simulink model "FastAndSlow"  (R2024b)
settings: Solver=VariableStepAuto  StartTime=0.0  StopTime=86400*2  RelTol=1e-3
values from neighbouring files (symbols this model uses):
  xk0 = zeros(36, 1)    [getinput_test.m]
(part 2 of 2)

== matlab function FastAndSlow/GP_1step ==
  data: y_model input; e_pred output; y_meas input; T input; P1 input; P2 input; P3 input; P4 input; P5 input; t input; comp_time output
function [e_pred, comp_time]= GP_onestep(y_model, y_meas, T, P1, P2, P3, P4, P5, t)
    
    % Declare we use some matlab function inside the Simulink block
    coder.extrinsic('fitrgp', 'predict')
    
    % Declare parameters
    n_regression = 4;
    sampling_time = 300;
    n_input = 6;
    n_output = size(y_model,1);
    delta_e_max = 20;
    n_max = 48; %300

    % Declare persistent variables whose dimension is not fixed (used to have an increasing dataset)
    persistent e_pers u_pers u_stack e_stack_1 e_stack_2 e_stack_3 e_stack_4 e_stack_5 e_stack_6 e_stack_7 e_stack_8 e_stack_9 e_stack_10 e_stack_11 e_stack_12 e_stack_13 e_stack_14 e_stack_15 e_stack_16 e_stack_17 e_pred_tot y_pers y_stack_1 y_stack_2 y_stack_3 y_stack_4 y_stack_5 y_stack_6 y_stack_7 y_stack_8 y_stack_9 y_stack_10 y_stack_11 y_stack_12 y_stack_13 y_stack_14 y_stack_15 y_stack_16 y_stack_17
    coder.varsize('u_pers', [inf, n_input]);
    coder.varsize('u_stack', [inf, n_input*n_regression]);
    coder.varsize('e_pred_tot', [inf, n_output]);
    coder.varsize('e_pers', [inf, n_output]);
    coder.varsize('e_stack_1', [inf, n_regression]);
    coder.varsize('e_stack_2', [inf, n_regression]);
    coder.varsize('e_stack_3', [inf, n_regression]);
    coder.varsize('e_stack_4', [inf, n_regression]);
    coder.varsize('e_stack_5', [inf, n_regression]);
    coder.varsize('e_stack_6', [inf, n_regression]);
    coder.varsize('e_stack_7', [inf, n_regression]);
    coder.varsize('e_stack_8', [inf, n_regression]);
    coder.varsize('e_stack_9', [inf, n_regression]);
    coder.varsize('e_stack_10', [inf, n_regression]);
    coder.varsize('e_stack_11', [inf, n_regression]);
    coder.varsize('e_stack_12', [inf, n_regression]);
    coder.varsize('e_stack_13', [inf, n_regression]);
    coder.varsize('e_stack_14', [inf, n_regression]);
    coder.varsize('e_stack_15', [inf, n_regression]);
    coder.varsize('e_stack_16', [inf, n_regression]);
    coder.varsize('e_stack_17', [inf, n_regression]);
    coder.varsize('y_pers', [inf, n_output]);
    coder.varsize('y_stack_1', [inf, n_regression]);
    coder.varsize('y_stack_2', [inf, n_regression]);
    coder.varsize('y_stack_3', [inf, n_regression]);
    coder.varsize('y_stack_4', [inf, n_regression]);
    coder.varsize('y_stack_5', [inf, n_regression]);
    coder.varsize('y_stack_6', [inf, n_regression]);
    coder.varsize('y_stack_7', [inf, n_regression]);
    coder.varsize('y_stack_8', [inf, n_regression]);
    coder.varsize('y_stack_9', [inf, n_regression]);
    coder.varsize('y_stack_10', [inf, n_regression]);
    coder.varsize('y_stack_11', [inf, n_regression]);
    coder.varsize('y_stack_12', [inf, n_regression]);
    coder.varsize('y_stack_13', [inf, n_regression]);
    coder.varsize('y_stack_14', [inf, n_regression]);
    coder.varsize('y_stack_15', [inf, n_regression]);
    coder.varsize('y_stack_16', [inf, n_regression]);
    coder.varsize('y_stack_17', [inf, n_regression]);
    
    % Initialize persistent variables
    if isempty(e_pers)
        u_pers = zeros(1,n_input);
        u_stack = zeros(1,n_input*n_regression);
        e_pred_tot = zeros(1,n_output);
        e_pers = zeros(1,n_output);
        e_stack_1 = zeros(1,n_regression);
        e_stack_2 = zeros(1,n_regression);
        e_stack_3 = zeros(1,n_regression);
        e_stack_4 = zeros(1,n_regression);
        e_stack_5 = zeros(1,n_regression);
        e_stack_6 = zeros(1,n_regression);
        e_stack_7 = zeros(1,n_regression);
        e_stack_8 = zeros(1,n_regression);
        e_stack_9 = zeros(1,n_regression);
        e_stack_10 = zeros(1,n_regression);
        e_stack_11 = zeros(1,n_regression);
        e_stack_12 = zeros(1,n_regression);
        e_stack_13 = zeros(1,n_regression);
        e_stack_14 = zeros(1,n_regression);
        e_stack_15 = zeros(1,n_regression);
        e_stack_16 = zeros(1,n_regression);
        e_stack_17 = zeros(1,n_regression);
        y_pers = zeros(1,n_output);
        y_stack_1 = zeros(1,n_regression);
        y_stack_2 = zeros(1,n_regression);
        y_stack_3 = zeros(1,n_regression);
        y_stack_4 = zeros(1,n_regression);
        y_stack_5 = zeros(1,n_regression);
        y_stack_6 = zeros(1,n_regression);
        y_stack_7 = zeros(1,n_regression);
        y_stack_8 = zeros(1,n_regression);
        y_stack_9 = zeros(1,n_regression);
        y_stack_10 = zeros(1,n_regression);
        y_stack_11 = zeros(1,n_regression);
        y_stack_12 = zeros(1,n_regression);
        y_stack_13 = zeros(1,n_regression);
        y_stack_14 = zeros(1,n_regression);
        y_stack_15 = zeros(1,n_regression);
        y_stack_16 = zeros(1,n_regression);
        y_stack_17 = zeros(1,n_regression);
    end
    
    % Output initialization
    e_pred = zeros(17,1);

    % Create increasing input dataset
    u_new = [T P1 P2 P3 P4 P5];
    u_pers = [u_pers; u_new];
    
    % Create increasing uncertainty dataset
    y_meas = [y_meas(1); y_meas(6); y_meas(11); y_meas(4); y_meas(9); y_meas(14); y_meas(2); y_meas(7); y_meas(12); y_meas(3); y_meas(8); y_meas(13); y_meas(5); y_meas(10); y_meas(15); y_meas(16); y_meas(17)];
    e_new = (y_meas - y_model).';
    e_pers = [e_pers; e_new];

    % Create increasing y model dataset
    y_pers = [y_pers; y_model.'];
    
    % Remove first row of zeros
    if e_pers(1,1) == 0
        u_pers = u_pers(2:end,:);
        e_pers = e_pers(2:end,:);
        y_pers = y_pers(2:end,:);
    end
    
    comp_time = 0;
    
    % Start to build GP when data are at least n_regression
    if t >= sampling_time*n_regression
        
        tic

        % Build the regressive variables
        u_regr = zeros(1,size(u_stack,2));
        u_regr_test = zeros(1,size(u_stack,2));
        k = 1;
        for i = 1:n_regression
            u_regr(1,k:k+n_input-1) = u_pers(end-i,:);
            u_regr_test(1,k:k+n_input-1) = u_pers(end-i+1,:);
            k = k + n_input;
        end

        e_regr_1 = zeros(1,size(e_stack_1,2));
        e_regr_1_test = zeros(1,size(e_stack_1,2));
        e_regr_2 = zeros(1,size(e_stack_2,2));
        e_regr_2_test = zeros(1,size(e_stack_2,2));
        e_regr_3 = zeros(1,size(e_stack_3,2));
        e_regr_3_test = zeros(1,size(e_stack_3,2));
        e_regr_4 = zeros(1,size(e_stack_4,2));
        e_regr_4_test = zeros(1,size(e_stack_4,2));
        e_regr_5 = zeros(1,size(e_stack_5,2));
        e_regr_5_test = zeros(1,size(e_stack_5,2));
        e_regr_6 = zeros(1,size(e_stack_6,2));
        e_regr_6_test = zeros(1,size(e_stack_6,2));
        e_regr_7 = zeros(1,size(e_stack_7,2));
        e_regr_7_test = zeros(1,size(e_stack_7,2));
        e_regr_8 = zeros(1,size(e_stack_8,2));
        e_regr_8_test = zeros(1,size(e_stack_8,2));
        e_regr_9 = zeros(1,size(e_stack_9,2));
        e_regr_9_test = zeros(1,size(e_stack_9,2));
        e_regr_10 = zeros(1,size(e_stack_10,2));
        e_regr_10_test = zeros(1,size(e_stack_10,2));
        e_regr_11 = zeros(1,size(e_stack_11,2));
        e_regr_11_test = zeros(1,size(e_stack_11,2));
        e_regr_12 = zeros(1,size(e_stack_12,2));
        e_regr_12_test = zeros(1,size(e_stack_12,2));
        e_regr_13 = zeros(1,size(e_stack_13,2));
        e_regr_13_test = zeros(1,size(e_stack_13,2));
        e_regr_14 = zeros(1,size(e_stack_14,2));
        e_regr_14_test = zeros(1,size(e_stack_14,2));
        e_regr_15 = zeros(1,size(e_stack_15,2));
        e_regr_15_test = zeros(1,size(e_stack_15,2));
        e_regr_16 = zeros(1,size(e_stack_16,2));
        e_regr_16_test = zeros(1,size(e_stack_16,2));
        e_regr_17 = zeros(1,size(e_stack_17,2));
        e_regr_17_test = zeros(1,size(e_stack_17,2));
        y_regr_1 = zeros(1,size(y_stack_1,2));
        y_regr_1_test = zeros(1,size(y_stack_1,2));
        y_regr_2 = zeros(1,size(y_stack_2,2));
        y_regr_2_test = zeros(1,size(y_stack_2,2));
        y_regr_3 = zeros(1,size(y_stack_3,2));
        y_regr_3_test = zeros(1,size(y_stack_3,2));
        y_regr_4 = zeros(1,size(y_stack_4,2));
        y_regr_4_test = zeros(1,size(y_stack_4,2));
        y_regr_5 = zeros(1,size(y_stack_5,2));
        y_regr_5_test = zeros(1,size(y_stack_5,2));
        y_regr_6 = zeros(1,size(y_stack_6,2));
        y_regr_6_test = zeros(1,size(y_stack_6,2));
        y_regr_7 = zeros(1,size(y_stack_7,2));
        y_regr_7_test = zeros(1,size(y_stack_7,2));
        y_regr_8 = zeros(1,size(y_stack_8,2));
        y_regr_8_test = zeros(1,size(y_stack_8,2));
        y_regr_9 = zeros(1,size(y_stack_9,2));
        y_regr_9_test = zeros(1,size(y_stack_9,2));
        y_regr_10 = zeros(1,size(y_stack_10,2));
        y_regr_10_test = zeros(1,size(y_stack_10,2));
        y_regr_11 = zeros(1,size(y_stack_11,2));
        y_regr_11_test = zeros(1,size(y_stack_11,2));
        y_regr_12 = zeros(1,size(y_stack_12,2));
        y_regr_12_test = zeros(1,size(y_stack_12,2));
        y_regr_13 = zeros(1,size(y_stack_13,2));
        y_regr_13_test = zeros(1,size(y_stack_13,2));
        y_regr_14 = zeros(1,size(y_stack_14,2));
        y_regr_14_test = zeros(1,size(y_stack_14,2));
        y_regr_15 = zeros(1,size(y_stack_15,2));
        y_regr_15_test = zeros(1,size(y_stack_15,2));
        y_regr_16 = zeros(1,size(y_stack_16,2));
        y_regr_16_test = zeros(1,size(y_stack_16,2));
        y_regr_17 = zeros(1,size(y_stack_17,2));
        y_regr_17_test = zeros(1,size(y_stack_17,2));

        for i = 1:n_regression
            e_regr_1(1,i) = e_pers(end-i,1);
            e_regr_1_test(1,i) = e_pers(end-i+1,1);
            e_regr_2(1,i) = e_pers(end-i,2);
            e_regr_2_test(1,i) = e_pers(end-i+1,2);
            e_regr_3(1,i) = e_pers(end-i,3);
            e_regr_3_test(1,i) = e_pers(end-i+1,3);
            e_regr_4(1,i) = e_pers(end-i,4);
            e_regr_4_test(1,i) = e_pers(end-i+1,4);
            e_regr_5(1,i) = e_pers(end-i,5);
            e_regr_5_test(1,i) = e_pers(end-i+1,5);
            e_regr_6(1,i) = e_pers(end-i,6);
            e_regr_6_test(1,i) = e_pers(end-i+1,6);
            e_regr_7(1,i) = e_pers(end-i,7);
            e_regr_7_test(1,i) = e_pers(end-i+1,7);
            e_regr_8(1,i) = e_pers(end-i,8);
            e_regr_8_test(1,i) = e_pers(end-i+1,8);
            e_regr_9(1,i) = e_pers(end-i,9);
            e_regr_9_test(1,i) = e_pers(end-i+1,9);
            e_regr_10(1,i) = e_pers(end-i,10);
            e_regr_10_test(1,i) = e_pers(end-i+1,10);
            e_regr_11(1,i) = e_pers(end-i,11);
            e_regr_11_test(1,i) = e_pers(end-i+1,11);
            e_regr_12(1,i) = e_pers(end-i,12);
            e_regr_12_test(1,i) = e_pers(end-i+1,12);
            e_regr_13(1,i) = e_pers(end-i,13);
            e_regr_13_test(1,i) = e_pers(end-i+1,13);
            e_regr_14(1,i) = e_pers(end-i,14);
            e_regr_14_test(1,i) = e_pers(end-i+1,14);
            e_regr_15(1,i) = e_pers(end-i,15);
            e_regr_15_test(1,i) = e_pers(end-i+1,15);
            e_regr_16(1,i) = e_pers(end-i,16);
            e_regr_16_test(1,i) = e_pers(end-i+1,16);
            e_regr_17(1,i) = e_pers(end-i,17);
            e_regr_17_test(1,i) = e_pers(end-i+1,17);
            y_regr_1(1,i) = y_pers(end-i,1);
            y_regr_1_test(1,i) = y_pers(end-i+1,1);
            y_regr_2(1,i) = y_pers(end-i,2);
            y_regr_2_test(1,i) = y_pers(end-i+1,2);
            y_regr_3(1,i) = y_pers(end-i,3);
            y_regr_3_test(1,i) = y_pers(end-i+1,3);
            y_regr_4(1,i) = y_pers(end-i,4);
            y_regr_4_test(1,i) = y_pers(end-i+1,4);
            y_regr_5(1,i) = y_pers(end-i,5);
            y_regr_5_test(1,i) = y_pers(end-i+1,5);
            y_regr_6(1,i) = y_pers(end-i,6);
            y_regr_6_test(1,i) = y_pers(end-i+1,6);
            y_regr_7(1,i) = y_pers(end-i,7);
            y_regr_7_test(1,i) = y_pers(end-i+1,7);
            y_regr_8(1,i) = y_pers(end-i,8);
            y_regr_8_test(1,i) = y_pers(end-i+1,8);
            y_regr_9(1,i) = y_pers(end-i,9);
            y_regr_9_test(1,i) = y_pers(end-i+1,9);
            y_regr_10(1,i) = y_pers(end-i,10);
            y_regr_10_test(1,i) = y_pers(end-i+1,10);
            y_regr_11(1,i) = y_pers(end-i,11);
            y_regr_11_test(1,i) = y_pers(end-i+1,11);
            y_regr_12(1,i) = y_pers(end-i,12);
            y_regr_12_test(1,i) = y_pers(end-i+1,12);
            y_regr_13(1,i) = y_pers(end-i,13);
            y_regr_13_test(1,i) = y_pers(end-i+1,13);
            y_regr_14(1,i) = y_pers(end-i,14);
            y_regr_14_test(1,i) = y_pers(end-i+1,14);
            y_regr_15(1,i) = y_pers(end-i,15);
            y_regr_15_test(1,i) = y_pers(end-i+1,15);
            y_regr_16(1,i) = y_pers(end-i,16);
            y_regr_16_test(1,i) = y_pers(end-i+1,16);
            y_regr_17(1,i) = y_pers(end-i,17);
            y_regr_17_test(1,i) = y_pers(end-i+1,17);
        end
    
        % Stack vertically
        u_stack = [u_stack; u_regr];
        e_stack_1 = [e_stack_1; e_regr_1];
        e_stack_2 = [e_stack_2; e_regr_2];
        e_stack_3 = [e_stack_3; e_regr_3];
        e_stack_4 = [e_stack_4; e_regr_4];
        e_stack_5 = [e_stack_5; e_regr_5];
        e_stack_6 = [e_stack_6; e_regr_6];
        e_stack_7 = [e_stack_7; e_regr_7];
        e_stack_8 = [e_stack_8; e_regr_8];
        e_stack_9 = [e_stack_9; e_regr_9];
        e_stack_10 = [e_stack_10; e_regr_10];
        e_stack_11 = [e_stack_11; e_regr_11];
        e_stack_12 = [e_stack_12; e_regr_12];
        e_stack_13 = [e_stack_13; e_regr_13];
        e_stack_14 = [e_stack_14; e_regr_14];
        e_stack_15 = [e_stack_15; e_regr_15];
        e_stack_16 = [e_stack_16; e_regr_16];
        e_stack_17 = [e_stack_17; e_regr_17];
        y_stack_1 = [y_stack_1; y_regr_1];
        y_stack_2 = [y_stack_2; y_regr_2];
        y_stack_3 = [y_stack_3; y_regr_3];
        y_stack_4 = [y_stack_4; y_regr_4];
        y_stack_5 = [y_stack_5; y_regr_5];
        y_stack_6 = [y_stack_6; y_regr_6];
        y_stack_7 = [y_stack_7; y_regr_7];
        y_stack_8 = [y_stack_8; y_regr_8];
        y_stack_9 = [y_stack_9; y_regr_9];
        y_stack_10 = [y_stack_10; y_regr_10];
        y_stack_11 = [y_stack_11; y_regr_11];
        y_stack_12 = [y_stack_12; y_regr_12];
        y_stack_13 = [y_stack_13; y_regr_13];
        y_stack_14 = [y_stack_14; y_regr_14];
        y_stack_15 = [y_stack_15; y_regr_15];
        y_stack_16 = [y_stack_16; y_regr_16];
        y_stack_17 = [y_stack_17; y_regr_17];
        
        %%%%%%%%%% Input of GP %%%%%%%%%%
        % x_1 = [e_stack_1 y_stack_1 u_stack];
        % x_2 = [e_stack_2 y_stack_2 u_stack];
        % x_3 = [e_stack_3 y_stack_3 u_stack];
        % x_4 = [e_stack_4 y_stack_4 u_stack];
        % x_5 = [e_stack_5 y_stack_5 u_stack];
        % x_6 = [e_stack_6 y_stack_6 u_stack];
        % x_7 = [e_stack_7 y_stack_7 u_stack];
        % x_8 = [e_stack_8 y_stack_8 u_stack];
        % x_9 = [e_stack_9 y_stack_9 u_stack];
        % x_10 = [e_stack_10 y_stack_10 u_stack];
        % x_11 = [e_stack_11 y_stack_11 u_stack];
        % x_12 = [e_stack_12 y_stack_12 u_stack];
        % x_13 = [e_stack_13 y_stack_13 u_stack];
        % x_14 = [e_stack_14 y_stack_14 u_stack];
        % x_15 = [e_stack_15 y_stack_15 u_stack];
        % x_16 = [e_stack_16 y_stack_16 u_stack];
        % x_17 = [e_stack_17 y_stack_17 u_stack];

        x_1 = [e_stack_1 y_stack_1];
        x_2 = [e_stack_2 y_stack_2];
        x_3 = [e_stack_3 y_stack_3];
        x_4 = [e_stack_4 y_stack_4];
        x_5 = [e_stack_5 y_stack_5];
        x_6 = [e_stack_6 y_stack_6];
        x_7 = [e_stack_7 y_stack_7];
        x_8 = [e_stack_8 y_stack_8];
        x_9 = [e_stack_9 y_stack_9];
        x_10 = [e_stack_10 y_stack_10];
        x_11 = [e_stack_11 y_stack_11];
        x_12 = [e_stack_12 y_stack_12];
        x_13 = [e_stack_13 y_stack_13];
        x_14 = [e_stack_14 y_stack_14];
        x_15 = [e_stack_15 y_stack_15];
        x_16 = [e_stack_16 y_stack_16];
        x_17 = [e_stack_17 y_stack_17];

        %%%%%%%%%% GP model learning, for each output %%%%%%%%%%
        gpr_model1 = fitrgp(x_1, e_pers(n_regression:end,1));
        gpr_model2 = fitrgp(x_2, e_pers(n_regression:end,2));
        gpr_model3 = fitrgp(x_3, e_pers(n_regression:end,3));
        gpr_model4 = fitrgp(x_4, e_pers(n_regression:end,4));
        gpr_model5 = fitrgp(x_5, e_pers(n_regression:end,5));
        gpr_model6 = fitrgp(x_6, e_pers(n_regression:end,6));
        gpr_model7 = fitrgp(x_7, e_pers(n_regression:end,7));
        gpr_model8 = fitrgp(x_8, e_pers(n_regression:end,8));
        gpr_model9 = fitrgp(x_9, e_pers(n_regression:end,9));
        gpr_model10 = fitrgp(x_10, e_pers(n_regression:end,10));
        gpr_model11 = fitrgp(x_11, e_pers(n_regression:end,11));
        gpr_model12 = fitrgp(x_12, e_pers(n_regression:end,12));
        gpr_model13 = fitrgp(x_13, e_pers(n_regression:end,13));
        gpr_model14 = fitrgp(x_14, e_pers(n_regression:end,14));
        gpr_model15 = fitrgp(x_15, e_pers(n_regression:end,15));
        gpr_model16 = fitrgp(x_16, e_pers(n_regression:end,16));
        gpr_model17 = fitrgp(x_17, e_pers(n_regression:end,17));
        
        %%%%%%%%%% GP prediction %%%%%%%%%%
        % e_pred(1) = predict(gpr_model1, [e_regr_1_test y_regr_1_test u_regr_test]);
        % e_pred(2) = predict(gpr_model2, [e_regr_2_test y_regr_2_test u_regr_test]);
        % e_pred(3) = predict(gpr_model3, [e_regr_3_test y_regr_3_test u_regr_test]);
        % e_pred(4) = predict(gpr_model4, [e_regr_4_test y_regr_4_test u_regr_test]);
        % e_pred(5) = predict(gpr_model5, [e_regr_5_test y_regr_5_test u_regr_test]);
        % e_pred(6) = predict(gpr_model6, [e_regr_6_test y_regr_6_test u_regr_test]);
        % e_pred(7) = predict(gpr_model7, [e_regr_7_test y_regr_7_test u_regr_test]);
        % e_pred(8) = predict(gpr_model8, [e_regr_8_test y_regr_8_test u_regr_test]);
        % e_pred(9) = predict(gpr_model9, [e_regr_9_test y_regr_9_test u_regr_test]);
        % e_pred(10) = predict(gpr_model10, [e_regr_10_test y_regr_10_test u_regr_test]);
        % e_pred(11) = predict(gpr_model11, [e_regr_11_test y_regr_11_test u_regr_test]);
        % e_pred(12) = predict(gpr_model12, [e_regr_12_test y_regr_12_test u_regr_test]);
        % e_pred(13) = predict(gpr_model13, [e_regr_13_test y_regr_13_test u_regr_test]);
        % e_pred(14) = predict(gpr_model14, [e_regr_14_test y_regr_14_test u_regr_test]);
        % e_pred(15) = predict(gpr_model15, [e_regr_15_test y_regr_15_test u_regr_test]);
        % e_pred(16) = predict(gpr_model16, [e_regr_16_test y_regr_16_test u_regr_test]);
        % e_pred(17) = predict(gpr_model17, [e_regr_17_test y_regr_17_test u_regr_test]);

        e_pred(1) = predict(gpr_model1, [e_regr_1_test y_regr_1_test]);
        e_pred(2) = predict(gpr_model2, [e_regr_2_test y_regr_2_test]);
        e_pred(3) = predict(gpr_model3, [e_regr_3_test y_regr_3_test]);
        e_pred(4) = predict(gpr_model4, [e_regr_4_test y_regr_4_test]);
        e_pred(5) = predict(gpr_model5, [e_regr_5_test y_regr_5_test]);
        e_pred(6) = predict(gpr_model6, [e_regr_6_test y_regr_6_test]);
        e_pred(7) = predict(gpr_model7, [e_regr_7_test y_regr_7_test]);
        e_pred(8) = predict(gpr_model8, [e_regr_8_test y_regr_8_test]);
        e_pred(9) = predict(gpr_model9, [e_regr_9_test y_regr_9_test]);
        e_pred(10) = predict(gpr_model10, [e_regr_10_test y_regr_10_test]);
        e_pred(11) = predict(gpr_model11, [e_regr_11_test y_regr_11_test]);
        e_pred(12) = predict(gpr_model12, [e_regr_12_test y_regr_12_test]);
        e_pred(13) = predict(gpr_model13, [e_regr_13_test y_regr_13_test]);
        e_pred(14) = predict(gpr_model14, [e_regr_14_test y_regr_14_test]);
        e_pred(15) = predict(gpr_model15, [e_regr_15_test y_regr_15_test]);
        e_pred(16) = predict(gpr_model16, [e_regr_16_test y_regr_16_test]);
        e_pred(17) = predict(gpr_model17, [e_regr_17_test y_regr_17_test]);

        
        %%%%%%%%%% Limit the difference of the uncertainty between two consecutive time instants %%%%%%%%%%
        for i = 1:n_output
            if abs(e_pred_tot(end,i)-e_pred(i)) > delta_e_max
                e_pred(i) = e_pred_tot(end,i);
            end
        end
       
        e_pred_tot = [e_pred_tot; e_pred.'];
    
        %%%%%%%%%% Limit the size of GP %%%%%%%%%%
        if size(u_stack,1) > n_max
            u_stack = u_stack(end-n_max:end,:);
            u_pers = u_pers(end-n_max-n_regression+1:end,:);
            e_pred_tot = e_pred_tot(end-n_max:end,:);
            e_pers = e_pers(end-n_max-n_regression+1:end,:);
            e_stack_1 = e_stack_1(end-n_max:end,:);
            e_stack_2 = e_stack_2(end-n_max:end,:);
            e_stack_3 = e_stack_3(end-n_max:end,:);
            e_stack_4 = e_stack_4(end-n_max:end,:);
            e_stack_5 = e_stack_5(end-n_max:end,:);
            e_stack_6 = e_stack_6(end-n_max:end,:);
            e_stack_7 = e_stack_7(end-n_max:end,:);
            e_stack_8 = e_stack_8(end-n_max:end,:);
            e_stack_9 = e_stack_9(end-n_max:end,:);
            e_stack_10 = e_stack_10(end-n_max:end,:);
            e_stack_11 = e_stack_11(end-n_max:end,:);
            e_stack_12 = e_stack_12(end-n_max:end,:);
            e_stack_13 = e_stack_13(end-n_max:end,:);
            e_stack_14 = e_stack_14(end-n_max:end,:);
            e_stack_15 = e_stack_15(end-n_max:end,:);
            e_stack_16 = e_stack_16(end-n_max:end,:);
            e_stack_17 = e_stack_17(end-n_max:end,:);
            y_pers = y_pers(end-n_max-n_regression+1:end,:);
            y_stack_1 = y_stack_1(end-n_max:end,:);
            y_stack_2 = y_stack_2(end-n_max:end,:);
            y_stack_3 = y_stack_3(end-n_max:end,:);
            y_stack_4 = y_stack_4(end-n_max:end,:);
            y_stack_5 = y_stack_5(end-n_max:end,:);
            y_stack_6 = y_stack_6(end-n_max:end,:);
            y_stack_7 = y_stack_7(end-n_max:end,:);
            y_stack_8 = y_stack_8(end-n_max:end,:);
            y_stack_9 = y_stack_9(end-n_max:end,:);
            y_stack_10 = y_stack_10(end-n_max:end,:);
            y_stack_11 = y_stack_11(end-n_max:end,:);
            y_stack_12 = y_stack_12(end-n_max:end,:);
            y_stack_13 = y_stack_13(end-n_max:end,:);
            y_stack_14 = y_stack_14(end-n_max:end,:);
            y_stack_15 = y_stack_15(end-n_max:end,:);
            y_stack_16 = y_stack_16(end-n_max:end,:);
            y_stack_17 = y_stack_17(end-n_max:end,:);
        end
       comp_time = toc
    end
end
